simulink library "ilcPerfIndx_cl"  (R2018b)
settings: Solver=VariableStepAuto  StartTime=0.0  StopTime=10.0  RelTol=1e-3
libraries: runningAvg_ul x1, stopwatch_ul x1
settings Model: Creator=mcobb  LastModifiedBy=mcobb

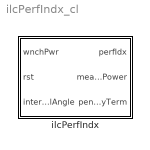
== system ilcPerfIndx_cl ==
  ilcPerfIndx : Subsystem  mask{w=0}
      mask prompts: w "Penalty Weight"

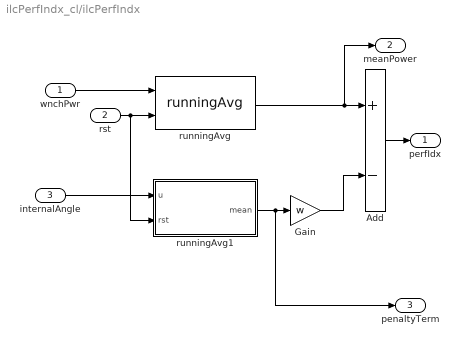
== system ilcPerfIndx_cl/ilcPerfIndx ==
  wnchPwr : Inport  PortDimensions=1
  rst : Inport  Port=2  PortDimensions=1
  internalAngle : Inport  Port=3  PortDimensions=1
  Add : Sum  Inputs=+-
  Gain : Gain  Gain=w
  runningAvg : runningAvg_ul/runningAvg  SystemSampleTime=-1
  runningAvg1 : Subsystem
  perfIdx : Outport  PortDimensions=1
  meanPower : Outport  Port=2  PortDimensions=1
  penaltyTerm : Outport  Port=3  PortDimensions=1
  wires:
  rst/1 -> runningAvg1/2(rst), runningAvg/2
  wnchPwr/1 -> runningAvg/1
  Add/1 -> perfIdx/1
  runningAvg/1 -> meanPower/1, Add/1
  internalAngle/1 -> runningAvg1/1(u)
  runningAvg1/1(mean) -> penaltyTerm/1, Gain/1
  Gain/1 -> Add/2

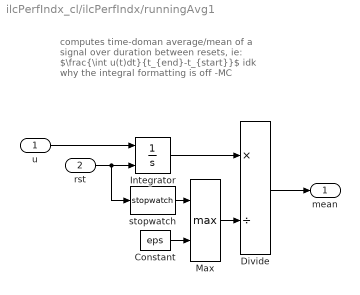
== system ilcPerfIndx_cl/ilcPerfIndx/runningAvg1 ==
  note: computes time-doman average/mean of a
      | signal over duration between resets, ie:
      | $\frac{\int u(t)dt}{t_{end}-t_{start}}$
      | idk why the integral formatting is off -MC
  u : Inport
  rst : Inport  Port=2
  Constant : Constant  Value=eps
  Divide : Product  Inputs=*/
  Integrator : Integrator  ExternalReset=rising
  Max : MinMax  Function=max  Inputs=2
  stopwatch : stopwatch_ul/stopwatch  SystemSampleTime=-1
  mean : Outport
  wires:
  Integrator/1 -> Divide/1
  u/1 -> Integrator/1
  stopwatch/1 -> Max/1
  Divide/1 -> mean/1
  Constant/1 -> Max/2
  Max/1 -> Divide/2
  rst/1 -> stopwatch/1, Integrator/2
